simulink model "Mathematical_Equation"  (R2019b)
settings: Solver=VariableStepAuto  StartTime=0.0  StopTime=10.0  RelTol=1e-3
values from neighbouring files (symbols this model uses):
  A = input(prompt1)    [Mathematical_Equation_Script.m]
  F = input(prompt)    [Mathematical_Equation_Script.m]
  Ti = input(prompt2)    [Mathematical_Equation_Script.m]
libraries: simulink x1
settings Model: Creator=Kudi Okerulu  LastModifiedBy=Kudi Okerulu

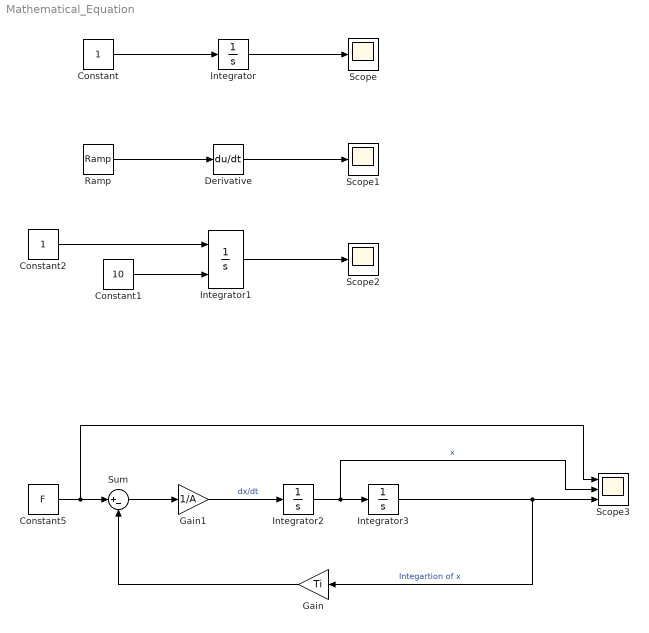
== system Mathematical_Equation ==
  Constant : Constant
  Constant1 : Constant  Value=10
  Constant2 : Constant
  Constant5 : Constant  Value=F
  Derivative : Derivative
  Gain : Gain  Gain=Ti
  Gain1 : Gain  Gain=1/A
  Integrator : Integrator
  Integrator1 : Integrator  InitialConditionSource=external  InitialCondition=2
  Integrator2 : Integrator
  Integrator3 : Integrator
  Ramp : simulink/Sources/Ramp  slope=1  start=0  InitialOutput=0
  Scope : Scope
  Scope1 : Scope
  Scope2 : Scope
  Scope3 : Scope  NumInputPorts=3
  Sum : Sum  Inputs=|+-
  wires:
  Constant/1 -> Integrator/1
  Integrator/1 -> Scope/1
  Derivative/1 -> Scope1/1
  Ramp/1 -> Derivative/1
  Integrator1/1 -> Scope2/1
  Constant1/1 -> Integrator1/2
  Constant2/1 -> Integrator1/1
  Integrator2/1 -> Scope3/2, Integrator3/1  "x"
  Sum/1 -> Gain1/1
  Integrator3/1 -> Scope3/3, Gain/1  "Integartion of x"
  Constant5/1 -> Scope3/1, Sum/1
  Gain/1 -> Sum/2
  Gain1/1 -> Integrator2/1  "dx/dt"
